simulink model "ASMC_interface"  (R2023b)
settings: Solver=ode4  StartTime=0.0  StopTime=10.0  FixedStep=0.01  RelTol=1e-3
undefined symbols (not defined in the file or in its folder): ArmConstants, ASMC, HexaConstants
settings Model: Creator=danie  LastModifiedBy=danie

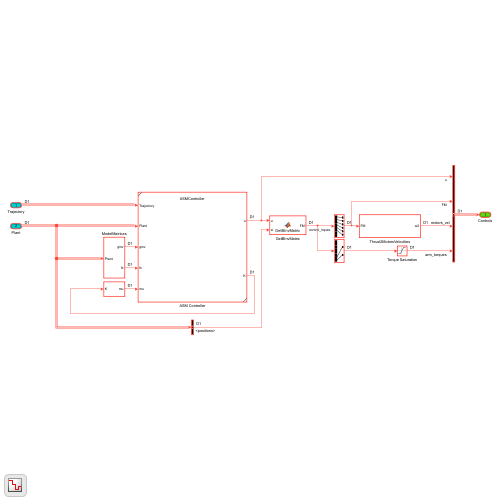
[thumbnail: Simulink's stored preview of the top-level diagram]
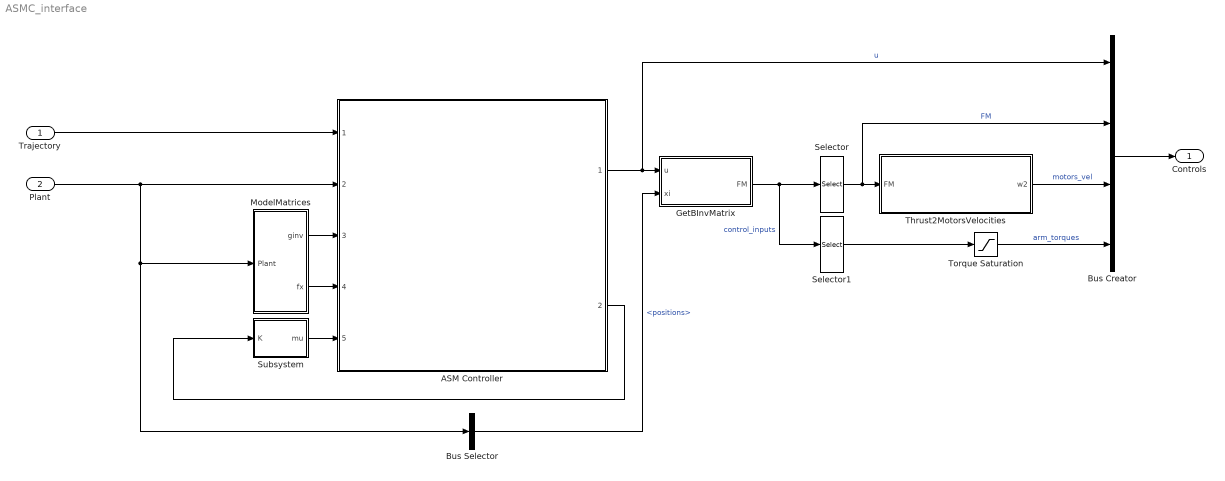
== system ASMC_interface ==
  Trajectory : Inport  OutDataTypeStr=Bus: TrajectoryBusDef  SampleTime=0.01
  Plant : Inport  Port=2  OutDataTypeStr=Bus: PlantBusDef  SampleTime=0.01
  ASM Controller : Subsystem  ReferencedSubsystem=ASMController
  Bus Creator : BusCreator  Inputs=4
  Bus Selector : BusSelector  OutputSignals=positions
  GetBInvMatrix : MATLAB Function  TreatAsAtomicUnit=on
  ModelMatrices : Subsystem
  Selector : Selector  InputPortWidth=8  IndexOptions=Index vector (dialog)  Indices=1:6  OutputSizes=1
  Selector1 : Selector  InputPortWidth=8  IndexOptions=Index vector (dialog)  Indices=7:8  OutputSizes=1
  Subsystem : Subsystem
  Thrust2MotorsVelocities : Subsystem
  Torque Saturation : Saturate  UpperLimit=ArmConstants.Servos.T1max  LowerLimit=-ArmConstants.Servos.T1max
  Controls : Outport  OutDataTypeStr=Bus: ControlsBusDef
  wires:
  Bus Selector/1 -> GetBInvMatrix/2(xi)  "<positions>"
  Subsystem/1(mu) -> ASM Controller/5
  Selector1/1 -> Torque Saturation/1
  ModelMatrices/2(fx) -> ASM Controller/4
  GetBInvMatrix/1(FM) -> Selector1/1, Selector/1  "control_inputs"
  ModelMatrices/1(ginv) -> ASM Controller/3
  Trajectory/1 -> ASM Controller/1
  Bus Creator/1 -> Controls/1
  Torque Saturation/1 -> Bus Creator/4  "arm_torques"
  ASM Controller/1 -> GetBInvMatrix/1(u), Bus Creator/1  "u"
  Plant/1 -> Bus Selector/1, ModelMatrices/1(Plant), ASM Controller/2
  Thrust2MotorsVelocities/1(w2) -> Bus Creator/3  "motors_vel"
  Selector/1 -> Bus Creator/2, Thrust2MotorsVelocities/1(FM)  "FM"
  ASM Controller/2 -> Subsystem/1(K)

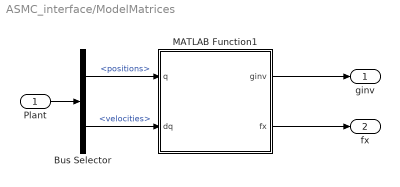
== system ASMC_interface/ModelMatrices ==
  Plant : Inport
  Bus Selector : BusSelector  OutputSignals=positions,velocities
  MATLAB Function1 : MATLAB Function  TreatAsAtomicUnit=on
  ginv : Outport
  fx : Outport  Port=2
  wires:
  Bus Selector/1 -> MATLAB Function1/1(q)  "<positions>"
  Bus Selector/2 -> MATLAB Function1/2(dq)  "<velocities>"
  Plant/1 -> Bus Selector/1
  MATLAB Function1/1(ginv) -> ginv/1
  MATLAB Function1/2(fx) -> fx/1

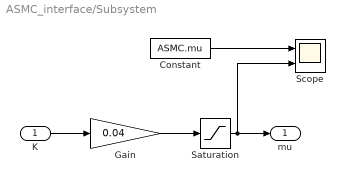
== system ASMC_interface/Subsystem ==
  K : Inport
  Constant : Constant  Value=ASMC.mu  SampleTime=-1
  Gain : Gain  Gain=0.04
  Saturation : Saturate  UpperLimit=ASMC.mu  LowerLimit=zeros(size(ASMC.mu))
  Scope : Scope  NumInputPorts=2
  mu : Outport
  wires:
  K/1 -> Gain/1
  Gain/1 -> Saturation/1
  Saturation/1 -> Scope/2, mu/1
  Constant/1 -> Scope/1

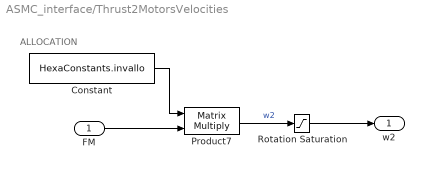
== system ASMC_interface/Thrust2MotorsVelocities ==
  note: ALLOCATION
  FM : Inport
  Constant : Constant  Value=HexaConstants.invallo  SampleTime=-1
  Product7 : Product  Multiplication=Matrix(*)
  Rotation Saturation : Saturate  UpperLimit=8.77e+05  LowerLimit=0
  w2 : Outport
  wires:
  FM/1 -> Product7/2
  Constant/1 -> Product7/1
  Product7/1 -> Rotation Saturation/1  "w2"
  Rotation Saturation/1 -> w2/1

== matlab function ASMC_interface/GetBInvMatrix ==
  data: u input; xi input; FM output
function FM = GetBInvMatrix(u,xi)

BM1 = BMatrix(xi);

BM = blkdiag(BM1, eye(2,2));

FM = BM\u;

end

== matlab function ASMC_interface/ModelMatrices/MATLAB Function1 ==
  data: q input; dq input; HexaConstants parameter; ginv output; fx output; ArmConstants parameter
function [ginv, fx] = Get_DCG_Hexa(q, dq, HexaConstants, ArmConstants)

DM = DMatrix(q, HexaConstants, ArmConstants);
CM = CMatrix(q, dq, HexaConstants, ArmConstants);
Gv = GVector(q, HexaConstants, ArmConstants);

ginv = DM;

fx = DM\( -CM*dq - Gv );

end
